simulink model "Demo2"  (R2019a)
settings: Solver=VariableStepAuto  StartTime=0.0  StopTime=1  RelTol=1e-3
settings Model: Creator=Admin  LastModifiedBy=Admin

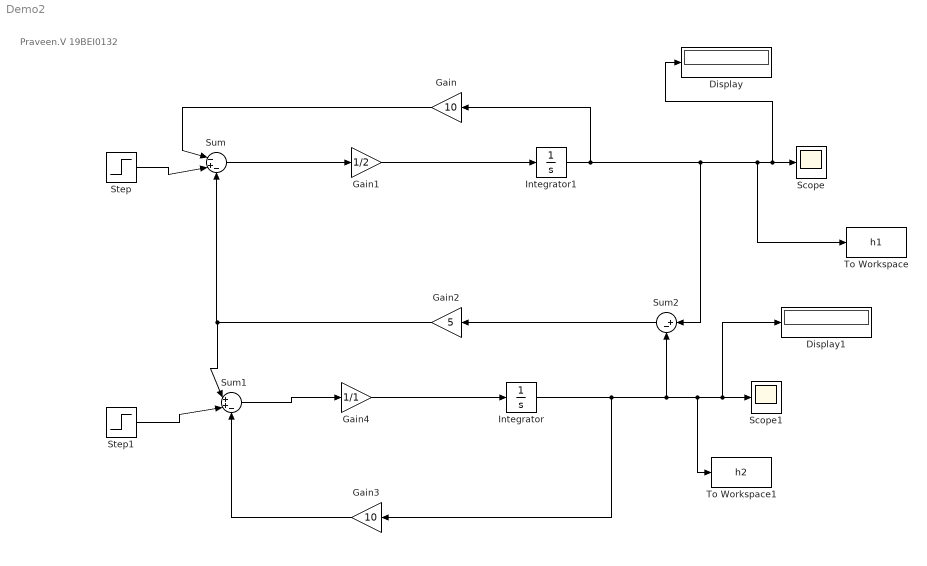
== system Demo2 ==
  note: Praveen.V
      | 19BEI0132
  Display : Display
  Display1 : Display
  Gain : Gain  Gain=10
  Gain1 : Gain  Gain=1/2
  Gain2 : Gain  Gain=5
  Gain3 : Gain  Gain=10
  Gain4 : Gain  Gain=1/1
  Integrator : Integrator
  Integrator1 : Integrator
  Scope : Scope
  Scope1 : Scope
  Step : Step  Time=0  SampleTime=0
  Step1 : Step  Time=0  SampleTime=0
  Sum : Sum  Inputs=|-+-
  Sum1 : Sum  Inputs=|++-
  Sum2 : Sum  Inputs=|+-
  To Workspace : ToWorkspace  VariableName=h1  SampleTime=-1
  To Workspace1 : ToWorkspace  VariableName=h2  SampleTime=-1
  wires:
  Gain4/1 -> Integrator/1
  Sum1/1 -> Gain4/1
  Sum2/1 -> Gain2/1
  Sum/1 -> Gain1/1
  Gain3/1 -> Sum1/3
  Step1/1 -> Sum1/2
  Step/1 -> Sum/2
  Gain2/1 -> Sum1/1, Sum/3
  Gain1/1 -> Integrator1/1
  Gain/1 -> Sum/1
  Integrator/1 -> Gain3/1, To Workspace1/1, Display1/1, Scope1/1, Sum2/2
  Integrator1/1 -> To Workspace/1, Display/1, Scope/1, Sum2/1, Gain/1
